simulink model "motorcontrol"  (R2020b)
settings: Solver=FixedStepDiscrete  StartTime=0.0  StopTime=20  FixedStep=Ts.simulink  MaxStep=5e-5  RelTol=1e-3  EnableMultiTasking=on
values from neighbouring files (symbols this model uses):
  dataType = 'single'    [motorcontrol_params.m]
undefined symbols (not defined in the file or in its folder): ControllerMode, ControlMode, ctrlParams, DiscIntNeverNeededParam, inverter, NumBits1, NumBits2, PI_params, pmsm, Slope1, Slope2, Ts
libraries: simulink x14, pid_lib x3
(part 3 of 3)

== system motorcontrol/Motor_Control4/Subsystem/Closed_Loop/Current_Controllers1/Subsystem ==
  Vd_ref : Inport
  Vq_ref : Inport  Port=2
  Data Type Duplicate : DataTypeDuplicate
  Demux : Demux  Outputs=2
  Gain : Gain  Gain=Vmax  OutDataTypeStr=Inherit: Same as input
  Math Function2 : Math  Operator=reciprocal  SignedPower=on  RndMeth=Simplest
  Mux : Mux  Inputs=2
  Product : Product  RndMeth=Simplest  OutDataTypeStr=Inherit: Same as first input
  Product1 : Product  RndMeth=Simplest  OutDataTypeStr=Inherit: Same as first input
  Product2 : Product  OutDataTypeStr=Inherit: Same as first input
  Sqrt : Sqrt  IntermediateResultsDataTypeStr=Inherit: Inherit from input  SaturateOnIntegerOverflow=on
  Sum2 : Sum  OutDataTypeStr=Inherit: Same as first input
  Switch : Switch  Threshold=Vmax  ZeroCross=off
  Vd_sat : Outport  VectorParamsAs1DForOutWhenUnconnected=off
  Vq_sat : Outport  Port=2  VectorParamsAs1DForOutWhenUnconnected=off
  wires:
  Vd_ref/1 -> Mux/1, Product/2, Product/1, Data Type Duplicate/1
  Demux/1 -> Vd_sat/1
  Product1/1 -> Sum2/2
  Product/1 -> Sum2/1
  Sum2/1 -> Sqrt/1
  Gain/1 -> Product2/1
  Math Function2/1 -> Gain/1
  Vq_ref/1 -> Mux/2, Product1/2, Product1/1, Data Type Duplicate/2
  Mux/1 -> Switch/3, Product2/2
  Product2/1 -> Switch/1
  Demux/2 -> Vq_sat/1
  Sqrt/1 -> Switch/2, Math Function2/1
  Switch/1 -> Demux/1

== system motorcontrol/Motor_Control4/Subsystem/Closed_Loop/Sine-Cosine Lookup/Subsystem ==
  In1 : Inport
  Compare To Zero : simulink/Logic and Bit Operations/Compare To Zero  relop=<  OutDataTypeStr=boolean
  Data Type Conversion : DataTypeConversion  OutDataTypeStr=uint16  ConvertRealWorld=Stored Integer (SI)  RndMeth=Simplest
  If : If
  Merge : Merge
  Subsystem : Subsystem
  Subsystem1 : Subsystem
  convert_pu : Gain  Gain=1/(dlgSett.UpperSatLimit)  RndMeth=Simplest  OutDataTypeStr=Inherit: Same as input
  Out1 : Outport
  wires:
  If/2 -> Subsystem1/Action
  Subsystem/1(Out1) -> Merge/1
  convert_pu/1 -> Subsystem1/1(In1), Subsystem/1(In1), Compare To Zero/1
  In1/1 -> convert_pu/1
  If/1 -> Subsystem/Action
  Subsystem1/1(Out1) -> Merge/2
  Data Type Conversion/1 -> If/1
  Compare To Zero/1 -> Data Type Conversion/1
  Merge/1 -> Out1/1

== system motorcontrol/Motor_Control4/Subsystem/Closed_Loop/Sine-Cosine Lookup/Subsystem1 ==
  In1 : Inport
  In2 : Inport  Port=2
  Demux : Demux
  Product : Product  RndMeth=Simplest  OutDataTypeStr=Inherit: Same as first input
  Product1 : Product  RndMeth=Simplest  OutDataTypeStr=Inherit: Same as first input
  Sum3 : Sum  Inputs=|+-  RndMeth=Simplest  OutDataTypeStr=Inherit: Same as first input
  Sum4 : Sum  Inputs=|++  RndMeth=Simplest  OutDataTypeStr=Inherit: Same as first input
  Sum5 : Sum  Inputs=|+-  RndMeth=Simplest  OutDataTypeStr=Inherit: Same as first input
  Sum6 : Sum  Inputs=|++  RndMeth=Simplest  OutDataTypeStr=Inherit: Same as first input
  Out1 : Outport
  Out2 : Outport  Port=2
  wires:
  Sum4/1 -> Out1/1
  Sum5/1 -> Product1/1
  Sum6/1 -> Out2/1
  Demux/1 -> Sum3/1
  Demux/2 -> Sum4/2, Sum3/2
  Product/1 -> Sum4/1
  Sum3/1 -> Product/1
  Product1/1 -> Sum6/1
  Demux/4 -> Sum5/2, Sum6/2
  In1/1 -> Demux/1
  Demux/3 -> Sum5/1
  In2/1 -> Product1/2, Product/2

== system motorcontrol/Motor_Control4/Subsystem/Closed_Loop/Subsystem3/Subsystem ==
  d : Inport
  q : Inport  Port=2
  D_axis_aligned : Mux  Inputs=2
  Demux : Demux  Outputs=2
  Offset : Constant  Value=dlgSett.Offset  OutDataTypeStr=uint16  SampleTime=-1
  Q_axis_aligned : Mux  Inputs=2
  Switch : Switch  Criteria=u2 > Threshold  Threshold=1  RndMeth=Simplest  ZeroCross=off
  Unary_Minus : UnaryMinus
  d_axis : Outport  VectorParamsAs1DForOutWhenUnconnected=off
  q_axis : Outport  Port=2  VectorParamsAs1DForOutWhenUnconnected=off
  wires:
  d/1 -> D_axis_aligned/1, Q_axis_aligned/2
  Demux/1 -> d_axis/1
  Switch/1 -> Demux/1
  Offset/1 -> Switch/2
  D_axis_aligned/1 -> Switch/3
  q/1 -> D_axis_aligned/2, Unary_Minus/1
  Q_axis_aligned/1 -> Switch/1
  Demux/2 -> q_axis/1
  Unary_Minus/1 -> Q_axis_aligned/1

== system motorcontrol/Motor_Control4/Subsystem/Closed_Loop/Subsystem4/Subsystem ==
  A : Inport
  B : Inport  Port=2
  D_axis_aligned : Mux  Inputs=2
  Demux : Demux  Outputs=2
  Offset : Constant  Value=dlgSett.Offset  OutDataTypeStr=uint16  SampleTime=-1
  Q_axis_aligned : Mux  Inputs=2
  Switch : Switch  Criteria=u2 > Threshold  Threshold=1  RndMeth=Simplest  ZeroCross=off
  Unary_Minus : UnaryMinus
  Alpha : Outport  VectorParamsAs1DForOutWhenUnconnected=off
  Beta : Outport  Port=2  VectorParamsAs1DForOutWhenUnconnected=off
  wires:
  Q_axis_aligned/1 -> Switch/1
  Demux/1 -> Alpha/1
  D_axis_aligned/1 -> Switch/3
  Switch/1 -> Demux/1
  A/1 -> Unary_Minus/1, D_axis_aligned/1
  Demux/2 -> Beta/1
  B/1 -> Q_axis_aligned/1, D_axis_aligned/2
  Offset/1 -> Switch/2
  Unary_Minus/1 -> Q_axis_aligned/2

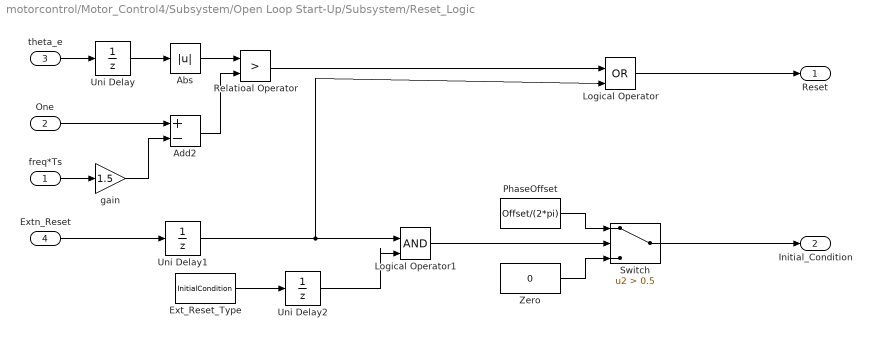
== system motorcontrol/Motor_Control4/Subsystem/Open Loop Start-Up/Subsystem/Reset_Logic ==
  freq*Ts : Inport
  One : Inport  Port=2
  theta_e : Inport  Port=3
  Extn_Reset : Inport  Port=4
  Abs : Abs  RndMeth=Simplest
  Add2 : Sum  Inputs=+-  RndMeth=Simplest  OutDataTypeStr=Inherit: Same as first input
  Ext_Reset_Type : Constant  Value=InitialCondition  OutDataTypeStr=boolean  SampleTime=-1
  Logical Operator : Logic  Operator=OR  IconShape=distinctive  AllPortsSameDT=off  OutDataTypeStr=boolean
  Logical Operator1 : Logic  IconShape=distinctive  AllPortsSameDT=off  OutDataTypeStr=boolean
  PhaseOffset : Constant  Value=Offset/(2*pi)  OutDataTypeStr=Inherit: Inherit via back propagation  SampleTime=-1
  Relatioal Operator : RelationalOperator  Operator=>  OutDataTypeStr=boolean  RndMeth=Simplest  InputSameDT=on
  Switch : Switch  Criteria=u2 > Threshold  Threshold=0.5  OutDataTypeStr=Inherit: Inherit via back propagation  RndMeth=Simplest
  Uni Delay : UnitDelay  SampleTime=-1  HasFrameUpgradeWarning=on
  Uni Delay1 : UnitDelay  InitialCondition=1  SampleTime=-1  HasFrameUpgradeWarning=on
  Uni Delay2 : UnitDelay  InitialCondition=1  SampleTime=-1  HasFrameUpgradeWarning=on
  Zero : Constant  Value=0  OutDataTypeStr=Inherit: Inherit via back propagation  SampleTime=-1
  gain : Gain  Gain=1.5  RndMeth=Simplest  OutDataTypeStr=Inherit: Same as input
  Reset : Outport  VectorParamsAs1DForOutWhenUnconnected=off
  Initial_Condition : Outport  Port=2  VectorParamsAs1DForOutWhenUnconnected=off
  wires:
  Uni Delay2/1 -> Logical Operator1/2
  theta_e/1 -> Uni Delay/1
  gain/1 -> Add2/2
  Logical Operator1/1 -> Switch/2
  Ext_Reset_Type/1 -> Uni Delay2/1
  freq*Ts/1 -> gain/1
  Logical Operator/1 -> Reset/1
  Uni Delay/1 -> Abs/1
  One/1 -> Add2/1
  Switch/1 -> Initial_Condition/1
  Relatioal Operator/1 -> Logical Operator/1
  Uni Delay1/1 -> Logical Operator/2, Logical Operator1/1
  Extn_Reset/1 -> Uni Delay1/1
  Add2/1 -> Relatioal Operator/2
  Zero/1 -> Switch/3
  PhaseOffset/1 -> Switch/1
  Abs/1 -> Relatioal Operator/1

== system motorcontrol/Motor_Control4/Subsystem/Open Loop Start-Up/Subsystem/Theta_IncrementSource ==
  In1 : Inport
  scale : Gain  Gain=1/(2*pi)  RndMeth=Simplest  OutDataTypeStr=Inherit: Same as input
  Out1 : Outport  VectorParamsAs1DForOutWhenUnconnected=off
  wires:
  In1/1 -> scale/1
  scale/1 -> Out1/1

== system motorcontrol/Motor_Control4/Subsystem/Open Loop Start-Up/Subsystem1/Sine-Cosine Lookup ==
  Theta : Inport
  Data Type Duplicate : DataTypeDuplicate  NumInputPorts=4
  Data Type Propagation : simulink/Signal Attributes/Data Type Propagation  PropDataType=fixdt(1, 16)  IfRefDouble=double  IfRefSingle=single  IsSigned=IsSigned1 or IsSigned2  NumBitsBase=max([NumBits1 NumBits2])  NumBitsMult=1  NumBitsAdd=0  NumBitsAllowFinal=1:128  PropScalingMode=Obtain via best precision  PropScaling=2^-10  ValuesUsedBestPrec=[0 dlgSett.index_gain]  SlopeBase=min([Slope1 Slope2])  SlopeMult=1  SlopeAdd=0  BiasBase=Bias1  BiasMult=1  BiasAdd=0
      settings: SourceProductBaseCode=SL
  Data Type Conversion1 : DataTypeConversion  RndMeth=Simplest
  Get_FractionVal : DataTypeConversion  RndMeth=Simplest
  Get_Integer : DataTypeConversion  OutDataTypeStr=uint16  RndMeth=Simplest
  Lookup : Selector  IndexMode=Zero-based  InputPortWidth=dlgSett.size  IndexOptions=Index vector (port)  Indices=[1 3]  OutputSizes=1
  Subsystem : Subsystem
  Subsystem1 : Subsystem
  Sum : Sum  Inputs=|++  AccumDataTypeStr=uint32  OutDataTypeStr=uint32  RndMeth=Simplest
  Sum2 : Sum  Inputs=|+-  RndMeth=Simplest  OutDataTypeStr=Inherit: Same as first input
  indexing : Gain  Gain=dlgSett.index_gain  OutDataTypeStr=Inherit: Inherit via back propagation  RndMeth=Simplest
  offset : Constant  Value=[1 0 (dlgSett.Offset+1) dlgSett.Offset]  OutDataTypeStr=int16  SampleTime=-1
  sine_table_values : Constant  Value=dlgSett.sin_table  OutDataTypeStr=Inherit: Inherit via back propagation  SampleTime=-1
  sin : Outport  VectorParamsAs1DForOutWhenUnconnected=off
  cos : Outport  Port=2  VectorParamsAs1DForOutWhenUnconnected=off
  wires:
  Subsystem1/2(Out2) -> cos/1
  Data Type Conversion1/1 -> Sum2/2
  Subsystem1/1(Out1) -> sin/1
  offset/1 -> Sum/2
  Lookup/1 -> Subsystem1/1(In1), Data Type Duplicate/3
  Get_FractionVal/1 -> Subsystem1/2(In2), Data Type Duplicate/4
  Sum/1 -> Lookup/2
  Theta/1 -> Subsystem/1(In1), Data Type Propagation/1, Data Type Propagation/2, Data Type Duplicate/1
  indexing/1 -> Get_Integer/1, Data Type Propagation/3, Sum2/1
  sine_table_values/1 -> Data Type Duplicate/2, Lookup/1
  Get_Integer/1 -> Data Type Conversion1/1, Sum/1
  Sum2/1 -> Get_FractionVal/1
  Subsystem/1(Out1) -> indexing/1

== system motorcontrol/Motor_Control4/Subsystem/Open Loop Start-Up/Subsystem1/Subsystem1 ==
  In1 : Inport
  In2 : Inport  Port=2
  Data Type Duplicate : DataTypeDuplicate
  add_b : Sum  Inputs=-+  RndMeth=Simplest  OutDataTypeStr=Inherit: Same as first input
  add_c : Sum  Inputs=--  RndMeth=Simplest  OutDataTypeStr=Inherit: Same as first input
  one_by_two : Gain  Gain=1/2  RndMeth=Simplest  OutDataTypeStr=Inherit: Same as input
  sqrt3_by_two : Gain  Gain=sqrt(3)/2  RndMeth=Simplest  OutDataTypeStr=Inherit: Same as input
  a : Outport  VectorParamsAs1DForOutWhenUnconnected=off
  b : Outport  Port=2  VectorParamsAs1DForOutWhenUnconnected=off
  c : Outport  Port=3  VectorParamsAs1DForOutWhenUnconnected=off
  wires:
  add_c/1 -> c/1
  one_by_two/1 -> add_b/1, add_c/1
  In2/1 -> sqrt3_by_two/1, Data Type Duplicate/2
  sqrt3_by_two/1 -> add_c/2, add_b/2
  add_b/1 -> b/1
  In1/1 -> one_by_two/1, Data Type Duplicate/1, a/1

== system motorcontrol/Motor_Control4/Subsystem/Open Loop Start-Up/Subsystem1/Subsystem2 ==
  Ds : Inport
  Qs : Inport  Port=2
  sin : Inport  Port=3
  cos : Inport  Port=4
  Data Type Duplicate : DataTypeDuplicate  NumInputPorts=4
  Subsystem : Subsystem
  dcos : Product  RndMeth=Simplest  OutDataTypeStr=Inherit: Same as first input
  dsin : Product  RndMeth=Simplest  OutDataTypeStr=Inherit: Same as first input
  qcos : Product  RndMeth=Simplest  OutDataTypeStr=Inherit: Same as first input
  qsin : Product  RndMeth=Simplest  OutDataTypeStr=Inherit: Same as first input
  sum_alpha : Sum  Inputs=|+-  RndMeth=Simplest  OutDataTypeStr=Inherit: Same as first input
  sum_beta : Sum  Inputs=|++  RndMeth=Simplest  OutDataTypeStr=Inherit: Same as first input
  Alpha : Outport  VectorParamsAs1DForOutWhenUnconnected=off
  Beta : Outport  Port=2  VectorParamsAs1DForOutWhenUnconnected=off
  wires:
  cos/1 -> qcos/2, dcos/2, Data Type Duplicate/3
  qsin/1 -> sum_alpha/2
  Subsystem/1(Alpha) -> Alpha/1
  Qs/1 -> qsin/1, qcos/1, Data Type Duplicate/2
  sum_beta/1 -> Subsystem/2(B)
  qcos/1 -> sum_beta/1
  dcos/1 -> sum_alpha/1
  Ds/1 -> dcos/1, dsin/1, Data Type Duplicate/1
  Subsystem/2(Beta) -> Beta/1
  sin/1 -> dsin/2, qsin/2, Data Type Duplicate/4
  sum_alpha/1 -> Subsystem/1(A)
  dsin/1 -> sum_beta/2

== system motorcontrol/Motor_Control1/PMSM/Subsystem/Subsystem/Subsystem2/Id cal ==
  Iq : Inport
  we : Inport  Port=2
  Vd : Inport  Port=3
  1/Ld : Gain  Gain=1/Ld  OutDataTypeStr=dataType  RndMeth=Simplest
  Constant : Constant  Value=idq0  OutDataTypeStr=single
  Constant1 : Constant  Value=2  OutDataTypeStr=single
  Discrete-Time Integrator3 : DiscreteIntegrator  InitialConditionSource=external  SampleTime=Ts  OutDataTypeStr=Inherit: Inherit via back propagation  LimitOutput=on  UpperSaturationLimit=10e6  LowerSaturationLimit=-10e6  ICPrevOutput=DiscIntNeverNeededParam  ICPrevScaledInput=DiscIntNeverNeededParam
  Index Vector : MultiPortSwitch  Inputs=1  OutDataTypeStr=Inherit: Inherit via back propagation
  Lq/Ld : Gain  Gain=Lq  OutDataTypeStr=dataType  RndMeth=Simplest
  Product : Product  RndMeth=Zero
  Rs/Ld : Gain  Gain=Rs  OutDataTypeStr=dataType  RndMeth=Simplest
  Sum : Sum  Inputs=-++
  Id : Outport
  wires:
  Iq/1 -> Product/1
  we/1 -> Product/2
  Product/1 -> Lq/Ld/1
  Discrete-Time Integrator3/1 -> Rs/Ld/1, Id/1
  Sum/1 -> 1/Ld/1
  Vd/1 -> Sum/3
  Lq/Ld/1 -> Sum/2
  Rs/Ld/1 -> Sum/1
  Constant/1 -> Index Vector/2
  Constant1/1 -> Index Vector/1
  1/Ld/1 -> Discrete-Time Integrator3/1
  Index Vector/1 -> Discrete-Time Integrator3/2

== system motorcontrol/Motor_Control1/PMSM/Subsystem/Subsystem/Subsystem2/Iq cal ==
  Id : Inport
  Vq : Inport  Port=2
  we : Inport  Port=3
  1/Lq : Gain  Gain=1/Lq  OutDataTypeStr=dataType  RndMeth=Simplest
  Constant : Constant  Value=idq0  OutDataTypeStr=single
  Constant1 : Constant  OutDataTypeStr=single
  Discrete-Time Integrator3 : DiscreteIntegrator  InitialConditionSource=external  SampleTime=Ts  OutDataTypeStr=Inherit: Inherit via back propagation  LimitOutput=on  UpperSaturationLimit=10e6  LowerSaturationLimit=-10e6  ICPrevOutput=DiscIntNeverNeededParam  ICPrevScaledInput=DiscIntNeverNeededParam
  Index Vector : MultiPortSwitch  Inputs=1  OutDataTypeStr=Inherit: Inherit via back propagation
  Ld/Lq : Gain  Gain=Ld  OutDataTypeStr=dataType  RndMeth=Simplest
  Product : Product  RndMeth=Zero
  Rs/Lq : Gain  Gain=Rs  OutDataTypeStr=dataType  RndMeth=Simplest
  Sum : Sum  Inputs=---+
  shi_f/Lq : Gain  Gain=FluxPM  OutDataTypeStr=dataType  RndMeth=Simplest
  Iq : Outport
  wires:
  Rs/Lq/1 -> Sum/1
  Ld/Lq/1 -> Sum/2
  shi_f/Lq/1 -> Sum/3
  Vq/1 -> Sum/4
  Sum/1 -> 1/Lq/1
  Discrete-Time Integrator3/1 -> Rs/Lq/1, Iq/1
  Product/1 -> Ld/Lq/1
  we/1 -> Product/2, shi_f/Lq/1
  Id/1 -> Product/1
  1/Lq/1 -> Discrete-Time Integrator3/1
  Constant/1 -> Index Vector/2
  Constant1/1 -> Index Vector/1
  Index Vector/1 -> Discrete-Time Integrator3/2

== system motorcontrol/Motor_Control4/Input Scaling/ Calculate Position and Speed/Subsystem3/Subsystem/Subsystem ==
  ϴm : Inport
  In2 : Inport  Port=2
  Action Port : ActionPort  ActionPortLabel=if(u1 <= u2)
  Add : Sum  Inputs=++-  RndMeth=Simplest  OutDataTypeStr=Inherit: Same as first input
  Constant : Constant  Value=maxAngleIn  OutDataTypeStr=Inherit: Inherit via back propagation
  Out1 : Outport
  wires:
  Add/1 -> Out1/1
  ϴm/1 -> Add/1
  Constant/1 -> Add/2
  In2/1 -> Add/3

== system motorcontrol/Motor_Control4/Input Scaling/ Calculate Position and Speed/Subsystem3/Subsystem/Subsystem1 ==
  ϴm : Inport
  In2 : Inport  Port=2
  Action Port : ActionPort  ActionPortLabel=else
  Add : Sum  Inputs=+-  RndMeth=Simplest  OutDataTypeStr=Inherit: Same as first input
  Out1 : Outport
  wires:
  Add/1 -> Out1/1
  ϴm/1 -> Add/1
  In2/1 -> Add/2

== system motorcontrol/Motor_Control4/Subsystem/Closed_Loop/Sine-Cosine Lookup/Subsystem/Subsystem ==
  In1 : Inport
  Action Port : ActionPort  ActionPortLabel=if(u1 > 0)
  Convert_back : DataTypeConversion  RndMeth=Simplest
  Convert_uint16 : DataTypeConversion  OutDataTypeStr=int16
  Data Type Duplicate : DataTypeDuplicate
  Sum : Sum  Inputs=|+-  RndMeth=Simplest  OutDataTypeStr=Inherit: Same as first input
  Out1 : Outport
  wires:
  In1/1 -> Data Type Duplicate/1, Sum/1, Convert_uint16/1
  Convert_uint16/1 -> Convert_back/1
  Convert_back/1 -> Sum/2, Data Type Duplicate/2
  Sum/1 -> Out1/1

== system motorcontrol/Motor_Control4/Subsystem/Closed_Loop/Sine-Cosine Lookup/Subsystem/Subsystem1 ==
  In1 : Inport
  Action Port : ActionPort  ActionPortLabel=else
  Convert_back : DataTypeConversion  RndMeth=Simplest
  Convert_uint16 : DataTypeConversion  OutDataTypeStr=int16  RndMeth=Simplest
  Data Type Duplicate : DataTypeDuplicate
  Sum : Sum  Inputs=|+-  RndMeth=Simplest  OutDataTypeStr=Inherit: Same as first input
  Out1 : Outport
  wires:
  Convert_uint16/1 -> Convert_back/1
  In1/1 -> Data Type Duplicate/1, Sum/1, Convert_uint16/1
  Convert_back/1 -> Sum/2, Data Type Duplicate/2
  Sum/1 -> Out1/1

== system motorcontrol/Motor_Control4/Subsystem/Open Loop Start-Up/Subsystem1/Sine-Cosine Lookup/Subsystem ==
  In1 : Inport
  Compare To Zero : simulink/Logic and Bit Operations/Compare To Zero  relop=<  OutDataTypeStr=boolean
  Data Type Conversion : DataTypeConversion  OutDataTypeStr=uint16  ConvertRealWorld=Stored Integer (SI)  RndMeth=Simplest
  If : If
  Merge : Merge
  Subsystem : Subsystem
  Subsystem1 : Subsystem
  convert_pu : Gain  Gain=1/(dlgSett.UpperSatLimit)  RndMeth=Simplest  OutDataTypeStr=Inherit: Same as input
  Out1 : Outport
  wires:
  If/2 -> Subsystem1/Action
  Subsystem/1(Out1) -> Merge/1
  convert_pu/1 -> Subsystem1/1(In1), Subsystem/1(In1), Compare To Zero/1
  In1/1 -> convert_pu/1
  If/1 -> Subsystem/Action
  Subsystem1/1(Out1) -> Merge/2
  Data Type Conversion/1 -> If/1
  Compare To Zero/1 -> Data Type Conversion/1
  Merge/1 -> Out1/1

== system motorcontrol/Motor_Control4/Subsystem/Open Loop Start-Up/Subsystem1/Sine-Cosine Lookup/Subsystem1 ==
  In1 : Inport
  In2 : Inport  Port=2
  Demux : Demux
  Product : Product  RndMeth=Simplest  OutDataTypeStr=Inherit: Same as first input
  Product1 : Product  RndMeth=Simplest  OutDataTypeStr=Inherit: Same as first input
  Sum3 : Sum  Inputs=|+-  RndMeth=Simplest  OutDataTypeStr=Inherit: Same as first input
  Sum4 : Sum  Inputs=|++  RndMeth=Simplest  OutDataTypeStr=Inherit: Same as first input
  Sum5 : Sum  Inputs=|+-  RndMeth=Simplest  OutDataTypeStr=Inherit: Same as first input
  Sum6 : Sum  Inputs=|++  RndMeth=Simplest  OutDataTypeStr=Inherit: Same as first input
  Out1 : Outport
  Out2 : Outport  Port=2
  wires:
  Sum4/1 -> Out1/1
  Sum5/1 -> Product1/1
  Sum6/1 -> Out2/1
  Demux/1 -> Sum3/1
  Demux/2 -> Sum4/2, Sum3/2
  Product/1 -> Sum4/1
  Sum3/1 -> Product/1
  Product1/1 -> Sum6/1
  Demux/4 -> Sum5/2, Sum6/2
  In1/1 -> Demux/1
  Demux/3 -> Sum5/1
  In2/1 -> Product1/2, Product/2

== system motorcontrol/Motor_Control4/Subsystem/Open Loop Start-Up/Subsystem1/Subsystem2/Subsystem ==
  A : Inport
  B : Inport  Port=2
  D_axis_aligned : Mux  Inputs=2
  Demux : Demux  Outputs=2
  Offset : Constant  Value=dlgSett.Offset  OutDataTypeStr=uint16  SampleTime=-1
  Q_axis_aligned : Mux  Inputs=2
  Switch : Switch  Criteria=u2 > Threshold  Threshold=1  RndMeth=Simplest  ZeroCross=off
  Unary_Minus : UnaryMinus
  Alpha : Outport  VectorParamsAs1DForOutWhenUnconnected=off
  Beta : Outport  Port=2  VectorParamsAs1DForOutWhenUnconnected=off
  wires:
  Unary_Minus/1 -> Q_axis_aligned/2
  Offset/1 -> Switch/2
  B/1 -> D_axis_aligned/2, Q_axis_aligned/1
  Demux/2 -> Beta/1
  A/1 -> D_axis_aligned/1, Unary_Minus/1
  Switch/1 -> Demux/1
  D_axis_aligned/1 -> Switch/3
  Demux/1 -> Alpha/1
  Q_axis_aligned/1 -> Switch/1

== system motorcontrol/Motor_Control4/Subsystem/Open Loop Start-Up/Subsystem1/Sine-Cosine Lookup/Subsystem/Subsystem ==
  In1 : Inport
  Action Port : ActionPort  ActionPortLabel=if(u1 > 0)
  Convert_back : DataTypeConversion  RndMeth=Simplest
  Convert_uint16 : DataTypeConversion  OutDataTypeStr=int16
  Data Type Duplicate : DataTypeDuplicate
  Sum : Sum  Inputs=|+-  RndMeth=Simplest  OutDataTypeStr=Inherit: Same as first input
  Out1 : Outport
  wires:
  In1/1 -> Data Type Duplicate/1, Sum/1, Convert_uint16/1
  Convert_uint16/1 -> Convert_back/1
  Convert_back/1 -> Sum/2, Data Type Duplicate/2
  Sum/1 -> Out1/1

== system motorcontrol/Motor_Control4/Subsystem/Open Loop Start-Up/Subsystem1/Sine-Cosine Lookup/Subsystem/Subsystem1 ==
  In1 : Inport
  Action Port : ActionPort  ActionPortLabel=else
  Convert_back : DataTypeConversion  RndMeth=Simplest
  Convert_uint16 : DataTypeConversion  OutDataTypeStr=int16  RndMeth=Simplest
  Data Type Duplicate : DataTypeDuplicate
  Sum : Sum  Inputs=|+-  RndMeth=Simplest  OutDataTypeStr=Inherit: Same as first input
  Out1 : Outport
  wires:
  Convert_uint16/1 -> Convert_back/1
  In1/1 -> Data Type Duplicate/1, Sum/1, Convert_uint16/1
  Convert_back/1 -> Sum/2, Data Type Duplicate/2
  Sum/1 -> Out1/1

== stateflow chart motorcontrol/Mode_Scheduler/Controller_Mode_Scheduler ==
  settings: updateMethod=DISCRETE  executeAtInitialization=1
  note: Controller Mode Scheduler
  note: The motor control algorithm begins in a stand-by mode awaiting a command to turn the motor on. Once this command
      | is issued the motor rotates to identify a known rotor position with valid position. The appropriate closed loop control then begins.
      | Upon a request to stop the motor, the motor will decellerate until zero speed is identified, after which the algorithm returns to the stand-by mode.
  state Stand_By
    entry: controller_mode = SpeedControl;
    velocity_command=0;
    torque_command = 0;
  state Motor_On
    state Motor_Control
      state Speed_Control
        entry: controller_mode = SpeedControl;
        en, du:
        velocity_command = command;
      state Position_Control
        entry: controller_mode = PositionControl;
        en,du:
        position_command = command;
      state Torque_Control
        entry: controller_mode = TorqueControl;
        en, du:
        torque_command = command;
      (default) -> (junction 386)
      (junction 386) -> Speed_Control [order 1] : [command_type==Speed]
      (junction 386) -> (junction 387) [order 2]
      (junction 387) -> Position_Control [order 1] : [command_type==Position]
      (junction 387) -> (junction 388) [order 2]
      (junction 388) -> Torque_Control : % [command_type==Torque]
  (default) -> Stand_By
  Stand_By -> Motor_On : [motor_on]
  Motor_On -> Stand_By : [~motor_on]
  data: controller_mode output Enum: ControllerMode; velocity_command output dataType; motor_on input boolean; position_command output dataType; command_type input Enum: ControlMode; torque_command output dataType; command input dataType

== matlab function motorcontrol/Motor_Control4/Subsystem/Closed_Loop/deadzone_comp ==
  settings: updateMethod=DISCRETE
  data: Ta output dataType; Tb output dataType; Tc output dataType; TaI input dataType; TbI input dataType; TcI input dataType
function [Ta,Tb,Tc] = deadzone_comp(TaI,TbI,TcI)
%#codegen

dbc = single(0.005);

if(TaI < 0)
    Ta = TaI - dbc;
elseif (TaI > 0)
    Ta = TaI + dbc;
else
    Ta = single(0);
end

if(TbI < 0)
    Tb = TbI - dbc;
elseif (TbI > 0)
    Tb = TbI + dbc;
else
    Tb = single(0);
end

if(TcI < 0)
    Tc = TcI - dbc;
elseif (TcI > 0)
    Tc = TcI + dbc;
else
    Tc = single(0);
end
